simulink model "export_data_from_simulink"  (R2024a)
settings: Solver=VariableStepAuto  StartTime=0.0  StopTime=10.0  MaxStep=1e-4  RelTol=1e-3
settings Model: Creator=admin  LastModifiedBy=admin

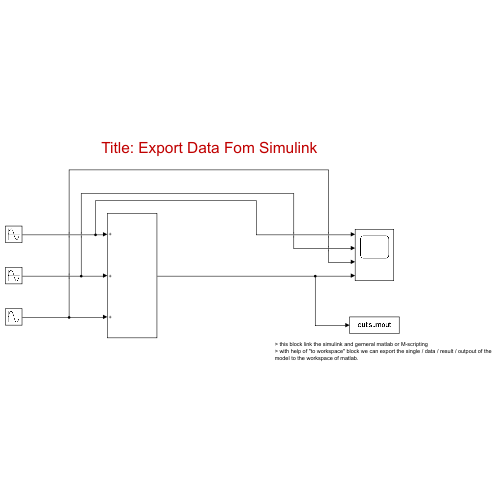
[thumbnail: Simulink's stored preview of the top-level diagram]
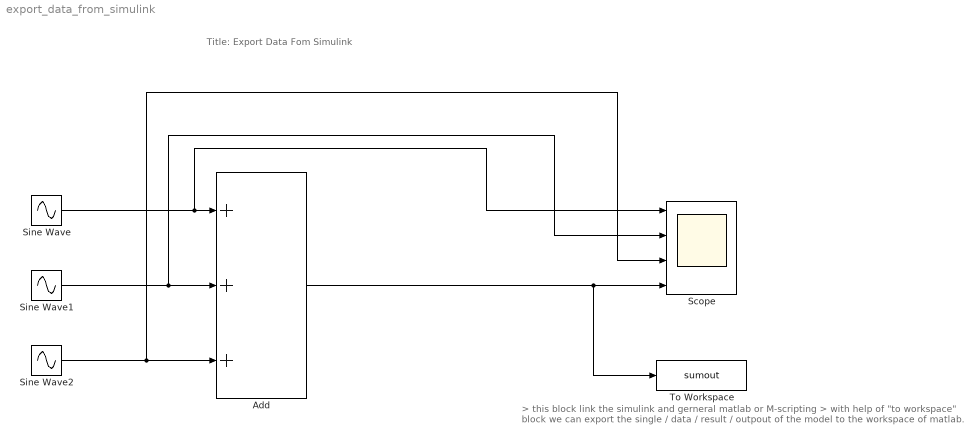
== system export_data_from_simulink ==
  note: Title: Export Data Fom Simulink
  note: > this block link the simulink and gerneral matlab or M-scripting
      | > with help of "to workspace" block we can export the single / data / result / outpout of the model to the workspace of matlab.
  Add : Sum  Inputs=+++
  Scope : Scope  NumInputPorts=4
  Sine Wave : Sin  SampleTime=0
  Sine Wave1 : Sin  Amplitude=2  SampleTime=0
  Sine Wave2 : Sin  Bias=1  Frequency=2  SampleTime=0
  To Workspace : ToWorkspace  VariableName=sumout  SaveFormat=Timeseries  SampleTime=-1
  wires:
  Sine Wave/1 -> Scope/1, Add/1
  Sine Wave2/1 -> Scope/3, Add/3
  Sine Wave1/1 -> Scope/2, Add/2
  Add/1 -> To Workspace/1, Scope/4
